simulink model "Plant_GasTurbine"  (R2012b)
settings: Solver=FixedStepDiscrete  StartTime=0.0  StopTime=MWS.in.SimTime  RelTol=1e-3
libraries: Lib_Turbo_Ambient_TMATS x1, Lib_Turbo_Burner_TMATS x1, Lib_Turbo_Compressor_TMATS x1, Lib_Turbo_Duct_TMATS x1, Lib_Turbo_Nozzle_TMATS x1, Lib_Turbo_Shaft_TMATS x1, Lib_Turbo_Turbine_TMATS x1
settings Model: Creator=jwchapm2  LastModifiedBy=jwchapm2
settings DataIOCC: SignalLoggingName=ILPlant
settings OptimizationCC: InlineParams=on

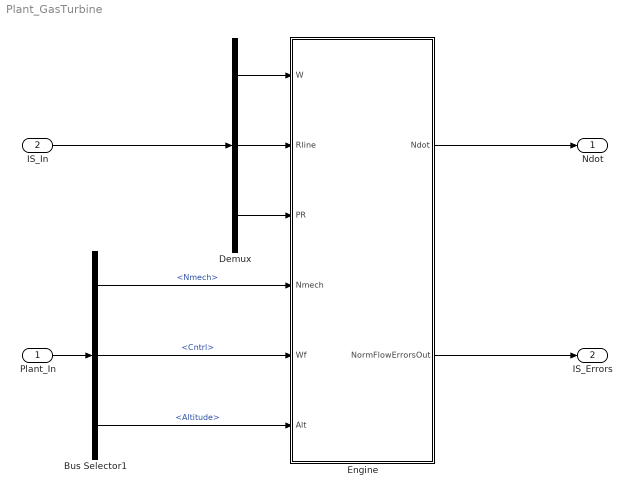
== system Plant_GasTurbine ==
  Plant_In : Inport  OutDataTypeStr=Bus: PlantInputs
  IS_In : Inport  Port=2
  Bus Selector1 : BusSelector  OutputSignals=OuterLoopPlantFeedback.Nmech,OuterLoopEffectors.Cntrl,OuterLoopEffectors.Altitude
  Demux : Demux  Outputs=3
  Engine : Subsystem
  Ndot : Outport
  IS_Errors : Outport  Port=2
  wires:
  Engine/2(NormFlowErrorsOut) -> IS_Errors/1
  Bus Selector1/2 -> Engine/5(Wf)  "<Cntrl>"
  Bus Selector1/1 -> Engine/4(Nmech)  "<Nmech>"
  Plant_In/1 -> Bus Selector1/1
  Engine/1(Ndot) -> Ndot/1
  Bus Selector1/3 -> Engine/6(Alt)  "<Altitude>"
  Demux/1 -> Engine/1(W)
  Demux/2 -> Engine/2(Rline)
  Demux/3 -> Engine/3(PR)
  IS_In/1 -> Demux/1

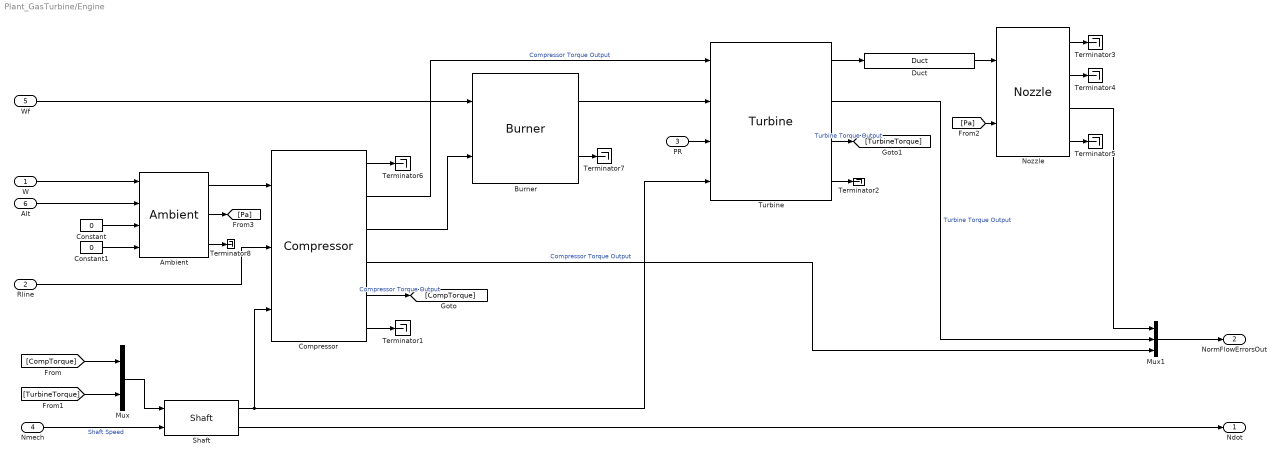
== system Plant_GasTurbine/Engine ==
  W : Inport
  Rline : Inport  Port=2
  PR : Inport  Port=3
  Nmech : Inport  Port=4
  Wf : Inport  Port=5
  Alt : Inport  Port=6
  Ambient : Lib_Turbo_Ambient_TMATS/Ambient  X_A_AltVec_M=5000*[-1 0 1 2 3 4 5 6 7 8 9 10 12 14 16]  T_A_TsVec_M=[536.51 518.67 500.84 483.03 465.22 447.41 429.62 411.84 394.06 389.97 389.97 389.97 389.97 392.25 397.69]  T_A_PsVec_M=[17.554 14.696 12.228 10.108 8.297 6.759 5.461 4.373 3.468 2.73 2.149 1.692 1.049 0.651 0.406]  AFARc_M=0
  Burner : Lib_Turbo_Burner_TMATS/Burner  LHV_M=MWS.Burner.LHV  dPnormBurner_M=MWS.Burner.dP
  Compressor : Lib_Turbo_Compressor_TMATS/Compressor  X_C_RlineVec_M=MWS.HPC.RlineVec  Y_C_NcVec_M=MWS.HPC.NcVec  T_C_Map_WcArray_M=MWS.HPC.WcArray  T_C_Map_PRArray_M=MWS.HPC.PRArray  T_C_Map_EffArray_M=MWS.HPC.EffArray  s_C_Nc_M=MWS.HPC.s_Nc  s_C_Wc_M=MWS.HPC.s_Wc  s_C_PR_M=MWS.HPC.s_PR  s_C_Eff_M=MWS.HPC.s_eff  CBLDEN_M=off  C_CBD_M=0  C_CBFht_M=0.5  C_CBFPt_M=0.5  FBLDEN_M=off  C_FBD_M=0  C_BFht_M=0.5  C_BFPt_M=0.5  X_C_WcSurgeVec_M=[0 200]  T_C_PRSurgeVec_M=[30 30]  iDesign_M=off  NcDes_M=10000  EffDes_M=0.95  PRDes_M=20  RlineDes_M=2
  Constant : Constant  Value=0
  Constant1 : Constant  Value=0
  Duct : Lib_Turbo_Duct_TMATS/Duct  dP_M=MWS.Duct.dP
  Mux : Mux  Inputs=2
  Mux1 : Mux  Inputs=3
  Nozzle : Lib_Turbo_Nozzle_TMATS/Nozzle  N_TArea_M=MWS.Noz.ATh  N_FL_M=MWS.Noz.LossPerc  X_N_TtVec2_M=MWS.Noz.TtVec  T_N_TGArray_M=MWS.Noz.TGArray  X_N_PEQPaVec_M=MWS.Noz.PeQPaVec  T_N_CdThArray_M=MWS.Noz.CdThArray  X_N_FARVec_M=MWS.Noz.FARVec  T_N_RtArray_M=MWS.Noz.RArray  Y_N_TtVec_M=MWS.Noz.TtVec  T_N_MAP_gammaArray_M=MWS.Noz.GArray  T_N_CvArray_M=MWS.Noz.CvArray  iDesign_M=off  WDes_M=100
  Shaft : Lib_Turbo_Shaft_TMATS/Shaft  Shaft_Inertia_M=MWS.Shaft.N_I
  Terminator{1..8} (8 alike) : Terminator
  Turbine : Lib_Turbo_Turbine_TMATS/Turbine  X_T_PRVec_M=MWS.HPT.PRVec  Y_T_NcVec_M=MWS.HPT.NcVec  T_T_Map_WcArray_M=MWS.HPT.WcArray  T_T_Map_EffArray_M=MWS.HPT.EffArray  s_T_Nc_M=MWS.HPT.s_Nc  s_T_PR_M=MWS.HPT.s_PR  s_T_Wc_M=MWS.HPT.s_Wc  s_T_Eff_M=MWS.HPT.s_eff  CFlwEn_M=off  T_CoolFlwPos_M=0  iDesign_M=off  NcDes_M=100  EffDes_M=0.9328  PRDes_M=5  NDes_M=10000
  Ndot : Outport
  NormFlowErrorsOut : Outport  Port=2
  wires:
  Compressor/3 -> Burner/2
  Wf/1 -> Burner/1
  Burner/2 -> Terminator7/1
  [Pa] -> Nozzle/2
  Burner/1 -> Turbine/2
  Turbine/1 -> Duct/1
  PR/1 -> Turbine/3
  Rline/1 -> Compressor/2
  Compressor/6 -> Terminator1/1
  Mux1/1 -> NormFlowErrorsOut/1
  Turbine/4 -> Terminator2/1
  Nozzle/1 -> Terminator3/1
  Nozzle/3 -> Mux1/1
  Nozzle/4 -> Terminator5/1
  Turbine/2 -> Mux1/2  "Turbine Torque Output"
  Compressor/4 -> Mux1/3  "Compressor Torque Output"
  Alt/1 -> Ambient/2
  Ambient/1 -> Compressor/1
  Nmech/1 -> Shaft/2  "Shaft Speed"
  Shaft/2 -> Ndot/1
  Mux/1 -> Shaft/1
  Compressor/5 -> [CompTorque]  "Compressor Torque Output"
  Turbine/3 -> [TurbineTorque]  "Turbine Torque Output"
  [CompTorque] -> Mux/1
  [TurbineTorque] -> Mux/2
  Shaft/1 -> Turbine/4, Compressor/3
  Compressor/1 -> Terminator6/1
  Compressor/2 -> Turbine/1  "Compressor Torque Output"
  Nozzle/2 -> Terminator4/1
  W/1 -> Ambient/1
  Constant/1 -> Ambient/3
  Constant1/1 -> Ambient/4
  Ambient/2 -> [Pa]
  Ambient/3 -> Terminator8/1
  Duct/1 -> Nozzle/1
